simulink model "convential"  (R2023b)
settings: Solver=ode23tb  StartTime=0.0  StopTime=1.5  RelTol=1e-3
model workspace (MAT data in the model file):
  F = Simulink.Parameter
  F.DataType = 'auto'
  F.Complexity = 'real'
  F.Dimensions = [0 0]
undefined symbols (not defined in the file or in its folder): sigbuilder_block
libraries: spsStairGeneratorLib x25, spsSeriesRLCBranchLib x3, simulink x3, spsDiodeLib x2, spsMosfetLib x1, spsPWMGeneratorDCDCLib x1, spsPVArrayLib x1, spsSeriesRLCLoadLib x1, sps_lib x1
settings Model: Creator=LOUZAZNI  LastModifiedBy=Hussein Sharadga
settings SolverCC: AlgebraicLoopSolver=TrustRegion
settings DebuggingCC: UnconnectedInputMsg=warning  UnconnectedOutputMsg=warning  UnconnectedLineMsg=warning  ArithmeticOperatorsInVariantConditions=warning
settings ModelReferenceCC: EnableRefExpFcnMdlSchedulingChecks=on
settings SFSimCC: CustomCodeUndefinedFunction=UseInterfaceOnly

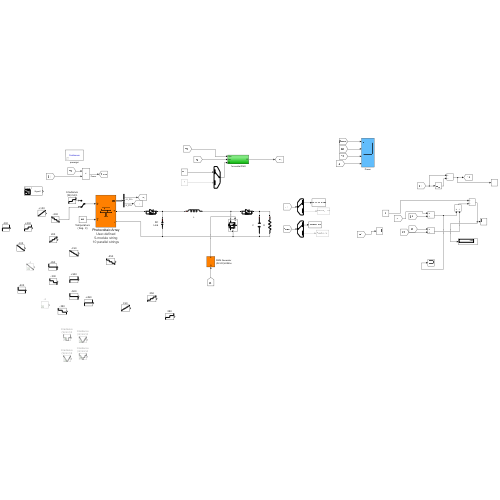
[thumbnail: Simulink's stored preview of the top-level diagram]
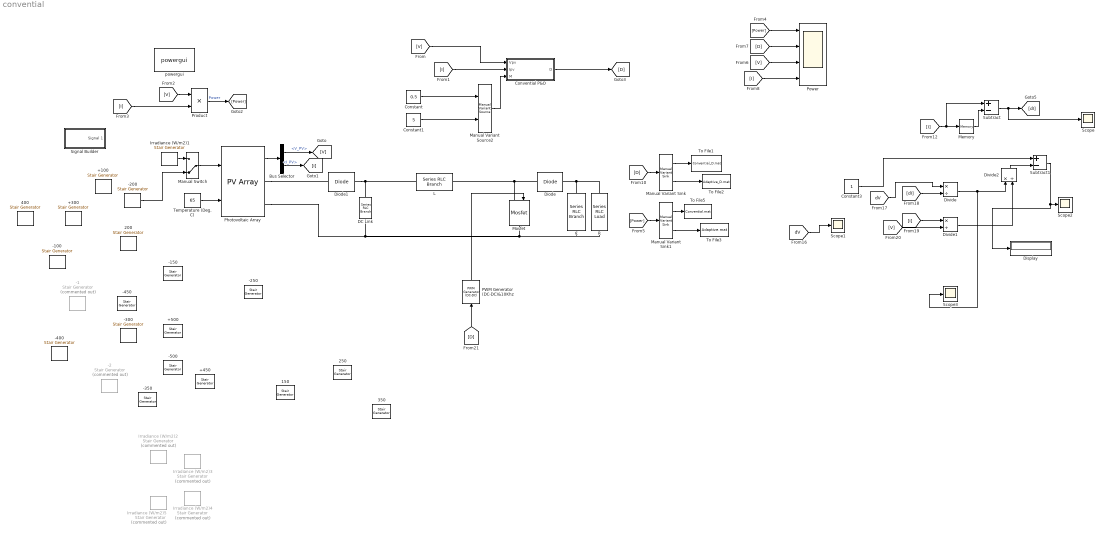
== system convential ==
  +100 : spsStairGeneratorLib/Stair Generator  t=[0,0.3,0.6,0.9,1.2,1.5,1.8,2.1,2.4]  e=[0.2,0.3,0.4,0.5,0.6,0.7,0.8,0.9,1]*1000  Ts=0.0001
  +300 : spsStairGeneratorLib/Stair Generator  t=[0,0.3,0.6,0.9]  e=[0.2,0.5,0.8,1.1]*1000  Ts=0.0001
  +450 : spsStairGeneratorLib/Stair Generator  t=[0, 0.3, 0.6]  e=[0.1,0.55, 1]*1000  Ts=0.0001
  +500 : spsStairGeneratorLib/Stair Generator  t=[0, 0.3, 0.6]  e=[0.1,0.6, 1.1]*1000  Ts=0.0001
  -1 : spsStairGeneratorLib/Stair Generator  Commented=on  t=[0,0.3,0.6,0.9,1.2,1.5,1.8,2.1,2.4,2.7,3,3.3,3.6,3.9,4.2,4.5,4.8,5.1,5.4]  e=[1.1,1.05,1,0.95,0.9,0.85,0.8,0.75,0.7,0.65,0.6,0.55,0.5,0.45,0.4,0.35,0.3,0.25,0.2]*1000  Ts=0.0001
  -100 : spsStairGeneratorLib/Stair Generator  t=[0,0.3,0.6,0.9,1.2,1.5,1.8,2.1,2.4]  e=[1,0.9,0.8,0.7,0.6,0.5,0.4,0.3,0.2]*1000  Ts=0.0001
  -150 : spsStairGeneratorLib/Stair Generator  t=[0, 0.3, 0.6, 0.9,1.2,1.5,1.8]  e=[1.1,0.95,0.8,0.65,0.5,0.35,0.2]*1000  Ts=0.0001
  -2 : spsStairGeneratorLib/Stair Generator  Commented=on  t=[0]  e=50  Ts=0.0001
  -200 : spsStairGeneratorLib/Stair Generator  t=[0,0.3,0.6,0.9,1.2]  e=[1,0.8,0.6,0.4,0.2]*1000  Ts=0.0001
  -250 : spsStairGeneratorLib/Stair Generator  t=[0, 0.3, 0.6, 0.9,1.2]  e=[1.1,0.85,0.6,0.35,0.1]*1000  Ts=0.0001
  -300 : spsStairGeneratorLib/Stair Generator  t=[0,0.3,0.6,0.9]  e=[1.1,0.8,0.5,0.2]*1000  Ts=0.0001
  -350 : spsStairGeneratorLib/Stair Generator  t=[0, 0.3, 0.6, 0.9]  e=[1.15,0.8,0.45,0.1]*1000  Ts=0.0001
  -400 : spsStairGeneratorLib/Stair Generator  t=[0,0.3,0.6]  e=[1,0.6,0.2]*1000  Ts=0.0001
  -450 : spsStairGeneratorLib/Stair Generator  t=[0, 0.3, 0.6]  e=[1,0.55,0.1]*1000  Ts=0.0001
  -500 : spsStairGeneratorLib/Stair Generator  t=[0, 0.3, 0.6]  e=[1.1,0.6,0.1]*1000  Ts=0.0001
  150 : spsStairGeneratorLib/Stair Generator  t=[0, 0.3, 0.6, 0.9,1.2,1.5,1.8]  e=[0.2,0.35, 0.5, 0.65,0.8,0.95,1.1]*1000  Ts=0.0001
  200 : spsStairGeneratorLib/Stair Generator  t=[0, 0.3, 0.6, 0.9,1.2]  e=[0.2,0.4, 0.6, 0.8,1]*1000  Ts=0.0001
  250 : spsStairGeneratorLib/Stair Generator  t=[0, 0.3, 0.6, 0.9,1.2]  e=[0.1,0.35, 0.6, 0.85,1.1]*1000  Ts=0.0001
  350 : spsStairGeneratorLib/Stair Generator  t=[0, 0.3, 0.6, 0.9]  e=[0.1,0.45, 0.8, 1.15]*1000  Ts=0.0001
  400 : spsStairGeneratorLib/Stair Generator  t=[0, 0.3, 0.6]  e=[0.2,0.6, 1]*1000  Ts=0.0001
  Bus Selector : BusSelector  OutputSignals=V_PV,I_PV
  C : spsSeriesRLCBranchLib/Series RLC Branch  LConnTagsString=__new0  RConnTagsString=__new0  BranchType=C  Resistance=1  Inductance=1e-3  SetiL0=off  InitialCurrent=0  Capacitance=50e-6  Setx0=off  InitialVoltage=600  Measurements=None
  Constant : Constant  Value=0.5
  Constant1 : Constant  Value=5
  Constant3 : Constant
  Convential P&O : Subsystem
  DC Link : spsSeriesRLCBranchLib/Series RLC Branch  LConnTagsString=__new0  RConnTagsString=__new0  BranchType=C  Resistance=0.001  Inductance=1.0  SetiL0=off  InitialCurrent=0  Capacitance=4000e-6  Setx0=off  InitialVoltage=310  Measurements=None
  Diode : spsDiodeLib/Diode  Ron=0.001  Lon=0  Vf=0.8  IC=0  UseSnubber=off  Rs=500  Cs=250e-9  Measurements=off
  Diode1 : spsDiodeLib/Diode  Ron=0.001  Lon=0  Vf=0.8  IC=0  UseSnubber=off  Rs=500  Cs=250e-9  Measurements=off
  Display : Display
  Divide : Product  Inputs=*/
  Divide1 : Product  Inputs=*/
  Divide2 : Product  Inputs=*/
  Irradiance (W/m2)1 : spsStairGeneratorLib/Stair Generator  t=[0, 0.3, 0.6, 0.9]  e=[0.2,0.5, 0.8, 1.1]*1000  Ts=0.0001
  Irradiance (W/m2)2 : spsStairGeneratorLib/Stair Generator  Commented=on  t=[0,0.3,0.6,0.9,1.2]  e=[1,0.6,0.2,0.6,1]*1000  Ts=0.0001
  Irradiance (W/m2)3 : spsStairGeneratorLib/Stair Generator  Commented=on  t=[0,0.3,0.6,0.9,1.2,1.5,1.8,2.1,2.4]  e=[1,0.8,0.6,0.4,0.2,0.4,0.6,0.8,1]*1000  Ts=0.0001
  Irradiance (W/m2)4 : spsStairGeneratorLib/Stair Generator  Commented=on  t=[0,0.3,0.6,0.9,1.2,1.5,1.8]  e=[1.1,0.8,0.5,0.2,0.5,0.8,1.1]*1000  Ts=0.0001
  Irradiance (W/m2)5 : spsStairGeneratorLib/Stair Generator  Commented=on  t=[0,0.3,0.6,0.9,1.2,1.5,1.8,2.1,2.4,2.7,3,3.3,3.6,3.9,4.2,4.5,4.8]  e=[1,0.9,0.8,0.7,0.6,0.5,0.4,0.3,0.2,0.3,0.4,0.5,0.6,0.7,0.8,0.9,1]*1000  Ts=0.0001
  L : spsSeriesRLCBranchLib/Series RLC Branch  LConnTagsString=__new0  RConnTagsString=__new0  BranchType=L  Resistance=0.01  Inductance=4e-4  SetiL0=off  InitialCurrent=5  Capacitance=1e-6  Setx0=off  InitialVoltage=0  Measurements=None
  Manual Variant Sink : simulink/Signal Routing/Manual Variant Sink  NumChoices=2  LabelModeActiveChoice=V_1
  Manual Variant Sink1 : simulink/Signal Routing/Manual Variant Sink  NumChoices=2  LabelModeActiveChoice=V_1
  Manual Variant Source2 : simulink/Signal Routing/Manual Variant Source  NumChoices=2  LabelModeActiveChoice=V_1
  Manual Switch : ManualSwitch  CurrentSetting=0
  Memory : Memory
  Mosfet : spsMosfetLib/Mosfet  Ron=0.1  Lon=0  Rd=0.01  Vfd=0  IC=0  Rs=1e5  Cs=inf  Measurements=off
  PWM Generator (DC-DC)&10Khz : spsPWMGeneratorDCDCLib/PWM Generator (DC-DC)  Fsw=5000  Ts=0
  Photovoltaic Array : spsPVArrayLib/PV Array  Npar=10  Nser=5  PlotType=one module @ 25 deg.C & specified irradiances  S_vec=[800]  Temp_C_vec=[ 50 ]  ModuleName=User-defined  PlotWhenSelected=off  Pm=210.16  Ncell=60  Voc=35.7  Isc=7.85  Vm=28.4  Im=7.4  beta_Voc_pc=-0.34  alpha_Isc_pc=0.041006  beta_Voc=-0.12138  alpha_Isc=0.003219  IL=7.8771  I0=1.268e-10  nI=0.93218  Rsh=515.1908  Rs=0.41772  RobustModel=off  RobustCellTemperature=313.3991  BAL=on  Tc=1e-6  Tfilter=5e-5
      settings: AttributesFormatString=|
      | %<ModuleName>
      | %<Nser>-module string
      | %<Npar> parallel strings
  Power : Scope  NumInputPorts=4
  Product : Product  RndMeth=Zero
  R : spsSeriesRLCLoadLib/Series RLC Load  LConnTagsString=a  RConnTagsString=__new0  NominalVoltage=30  NominalFrequency=50  ActivePower=120  InductivePower=0  CapacitivePower=0  Setx0=off  InitialVoltage=0  SetiL0=off  InitialCurrent=0  Measurements=None  LoadType=constant Z
  Scope{,1..3} (4 alike) : Scope
  Signal Builder : Subsystem  Tag=STV Subsys  LoadFcn=sigbuilder_block('load');  StartFcn=sigbuilder_block('start');  StopFcn=sigbuilder_block('stop');  ClipboardFcn=sigbuilder_block('clipboard');  mask(Sigbuilder block){tuvar=[0:10]}
      mask help: Simulink:masks:SigbuilderBlock_MD
      mask init:
      | if ~strcmp(get_param(bdroot(gcbh),'SimulationStatus'),'stopped') tuvar = sigbuilder_block('maskInit'); end
      settings: CopyFcn=sigbuilder_block('copy');  DeleteFcn=sigbuilder_block('delete');  ModelCloseFcn=sigbuilder_block('modelClose');  PreSaveFcn=sigbuilder_block('preSave');  PauseFcn=sigbuilder_block('pause');  ContinueFcn=sigbuilder_block('continue');  NameChangeFcn=sigbuilder_block('namechange');  OpenFcn=sigbuilder_block('open',[437.6 199.2 550.4 400 ]);  CloseFcn=sigbuilder_block('close');
      mask Display: plot(0, 0, 100, 100,[2, 2, 32, 32, 2], [68, 8, 8, 68, 68],[32, 2], [38, 38], [32, 19, 2],[53, 60, 44], [32, 17, 17, 2],[16, 16, 31, 31]);txt = getActiveGroup(gcbh);text(2, 100, txt,'verticalAlignment', 'top');
  Subtract : Sum  Inputs=+-
  Subtract1 : Sum  Inputs=+-
  Temperature (Deg. C) : Constant  Value=65
  To File1 : ToFile  Filename=Convential_D.mat  MatrixName=Convential_D  SaveFormat=Timeseries
  To File2 : ToFile  Filename=Adaptive_D.mat  MatrixName=Adaptive_D  SaveFormat=Timeseries
  To File3 : ToFile  Filename=Adaptive.mat  MatrixName=Adaptive  SaveFormat=Timeseries
  To File5 : ToFile  Filename=Convential.mat  MatrixName=Convential  SaveFormat=Timeseries
  powergui : sps_lib/powergui  Priority=1  SimulationMode=Continuous  SampleTime=5e-7  frequency=60  Iterations=50  frequencyindice=0  Pbase=100e6  ErrMax=1e-4  UnitsV=kV  UnitsW=MW  buscounter=0  FunctionMessages=off  echomessages=off  EnableUseOfTLC=off  CurrentSourceSwitches=off  DisableSnubberDevices=off  DisableRonSwitches=off  DisableVfSwitches=off  DisplayEquations=off  AutomaticDiscreteSolvers=off  SolverType=Tustin/Backward Euler (TBE)  Interpol=off  ExternalGateDelay=off  methode=off  Ts=100  x0status=blocks  SPID=off  SwTol=0  HookPort=off  NonlinearTolerance=1e-4  nMaxIteration=100  ContinueOnMaxIteration=off  RestoreLinks=warning  ResistiveCurrentMeasurement=off  Frange=[0:2:500]  Ylog=off  Xlog=on  ShowGrid=off  save=off  variable=ZData  structure=0  ZoomFFT=off  StartTime=0.0  cycles=1  DisplayStyle=1  fundamental=60  FreqAxis=off  MaxFrequency=1000  frequencyindicesteady=1  RmsSteady=1  display=off
  wires:
  Photovoltaic Array/1 -> Bus Selector/1
  Temperature (Deg. C)/1 -> Photovoltaic Array/2
  [V] -> Convential P&O/1(Vpv)
  [I] -> Convential P&O/2(Ipv)
  Bus Selector/1 -> [V]  "<V_PV>"
  Bus Selector/2 -> [I]  "<I_PV>"
  [V] -> Product/1
  [I] -> Product/2
  Manual Variant Sink/2 -> To File2/1
  Manual Variant Sink1/2 -> To File3/1
  Irradiance (W/m2)1/1 -> Manual Switch/1
  Manual Switch/1 -> Photovoltaic Array/1
  Manual Variant Sink1/1 -> To File5/1
  Product/1 -> [Power]  "Power"
  [Power] -> Power/1
  [Power] -> Manual Variant Sink1/1
  [V] -> Power/3
  [D] -> Power/2
  [D] -> Manual Variant Sink/1
  Manual Variant Sink/1 -> To File1/1
  Manual Variant Source2/1 -> Convential P&O/3(M)
  Constant/1 -> Manual Variant Source2/1
  Constant1/1 -> Manual Variant Source2/2
  [dV] -> Scope1/1
  [I] -> Divide1/1
  [V] -> Divide1/2
  Constant3/1 -> Subtract1/1
  Divide2/1 -> Subtract1/2
  Subtract1/1 -> Display/1, Scope2/1
  Divide1/1 -> Divide2/2
  Divide/1 -> Scope3/1, Divide2/1
  Memory/1 -> Subtract/2
  [I] -> Subtract/1, Memory/1
  Subtract/1 -> Scope/1, [dI]
  [D] -> PWM Generator (DC-DC)&10Khz/1
  PWM Generator (DC-DC)&10Khz/1 -> Mosfet/1
  Convential P&O/1(D) -> [D]
  [dI] -> Divide/2
  [dV] -> Divide/1
  [I] -> Power/4
  -200/1 -> Manual Switch/2
  connections:
  Photovoltaic Array/RConn2 -- DC Link/RConn1 -- Mosfet/RConn1 -- R/RConn1 -- C/RConn1
  Mosfet/LConn1 -- L/RConn1 -- Diode/LConn1
  Diode1/RConn1 -- DC Link/LConn1 -- L/LConn1
  C/LConn1 -- R/LConn1 -- Diode/RConn1
  Photovoltaic Array/RConn1 -- Diode1/LConn1

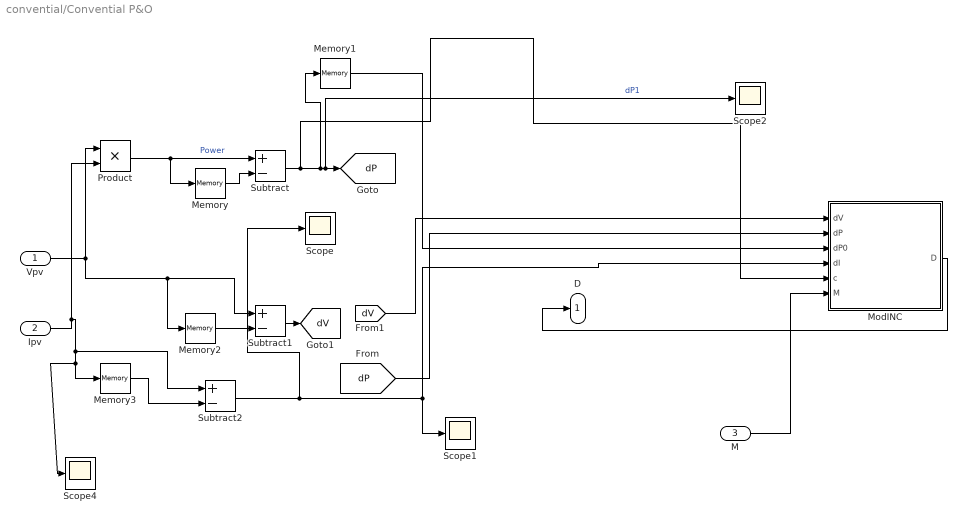
== system convential/Convential P&O ==
  Vpv : Inport
  Ipv : Inport  Port=2
  M : Inport  Port=3
  Memory : Memory
  Memory1 : Memory  InitialCondition=1
  Memory2 : Memory
  Memory3 : Memory
  ModINC : MATLAB Function  TreatAsAtomicUnit=on
  Product : Product
  Scope{,1..2,4} (4 alike) : Scope
  Subtract : Sum  Inputs=+-
  Subtract1 : Sum  Inputs=+-
  Subtract2 : Sum  Inputs=+-
  D : Outport  VectorParamsAs1DForOutWhenUnconnected=off
  tag scope: dP=global, dV=global
  wires:
  Subtract2/1 -> Scope1/1, ModINC/4(dI), Scope/1
  Memory3/1 -> Subtract2/2
  Memory1/1 -> ModINC/3(dP0)
  Subtract/1 -> Scope2/1, [dP], Memory1/1, ModINC/5(c)  "dP1"
  Ipv/1 -> Product/2, Memory3/1, Scope4/1, Subtract2/1
  [dV] -> ModINC/1(dV)
  Subtract1/1 -> [dV]
  Memory2/1 -> Subtract1/2
  [dP] -> ModINC/2(dP)
  Memory/1 -> Subtract/2
  Product/1 -> Subtract/1, Memory/1  "Power"
  ModINC/1(D) -> D/1
  Vpv/1 -> Product/1, Memory2/1, Subtract1/1
  M/1 -> ModINC/6(M)

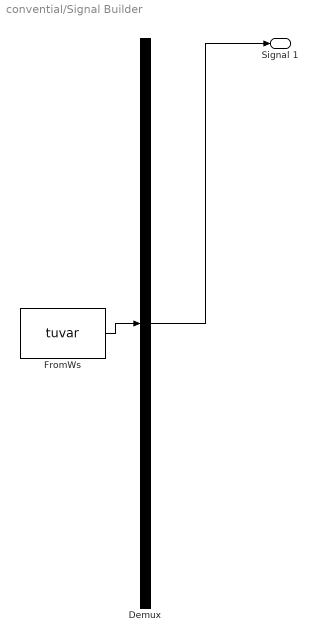
== system convential/Signal Builder ==
  Demux : Demux  Tag=STV Demux  Outputs=1
      settings: DisplayOption=none
  FromWs : FromWorkspace  Tag=STV FromWs  VariableName=tuvar
      SigBuilderData=|
      | common.afterFinalStr = 'Extrapolate'
      | common.sampleTime = 0
      | dataSet.timeRange = [0 1.8]
      | dataSet.name = 'Group 1'
      | sbobj.Groups.Name = 'Group 1'
      | sbobj.Groups.Signals.Name = 'Signal 1'
      | sbobj.Groups.Signals.XData = [0 0.3 0.6 0.9 1.2 1.8]
      | sbobj.Groups.Signals.YData = [1000 1000 600 600 1100 1100]
      | sbobj.Groups.TimeRange = [0 1.8]
  Signal 1 : Outport  Tag=STV Outport  VectorParamsAs1DForOutWhenUnconnected=off
  wires:
  Demux/1 -> Signal 1/1
  FromWs/1 -> Demux/1

== matlab function convential/Convential P&O/ModINC ==
  settings: updateMethod=DISCRETE
  data: D output; dV input; dP input; dP0 input; dI input; c input; M input

function D =ModINC(dV,dP,dP0,dI,c,M)


Dinit = 0.6;  %Initial value for D output
Dmax = 0.65;   %Maximum value for D
Dmin = 0;   %Minimum value for D
    deltaD = 0.0005;
   

persistent   Dold  ;


dataType = 'double';

if isempty(Dold)

    Dold=Dinit;
end
  
if dP == 0
                    D=Dold;
else
       if dP >0        
                        if dV>0
            D=Dold - M*deltaD;
            else
                            D=Dold + M*deltaD;
                        end
        else
                        if dV>0
            D=Dold + M*deltaD;
            else
                            D=Dold - M*deltaD;
                        end       
    end    
        
       
end

if D >= Dmax | D<= Dmin
    D=Dold;
end

Dold=D;
